simulink library "csu_und_unduplicate_lib"  (R2014b)
settings: Solver=ode45  SolverMode=SingleTasking  StartTime=0.0  StopTime=10.0  RelTol=1e-3
libraries: util_info_lib x1
settings Model: ExtModeAutoUpdateStatusClock=off  Creator=Administrator  LastModifiedBy=mstewart

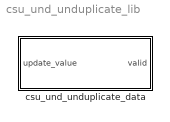
== system csu_und_unduplicate_lib ==
  csu_und_unduplicate_data : Subsystem  mask{initial_compare=0}
      mask prompts: initial_compare "initial comparison value"
      mask Display:
      | port_label('input',1,'update');
      | port_label('output',1','valid');

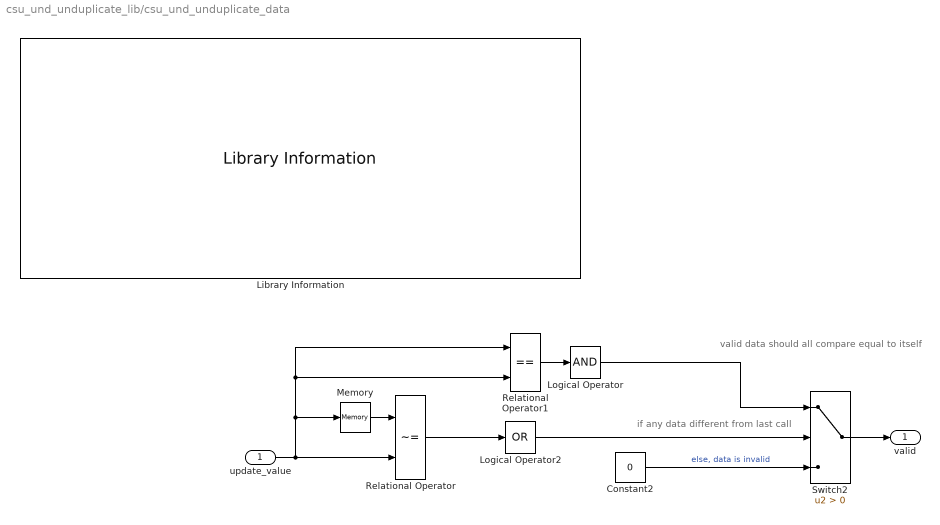
== system csu_und_unduplicate_lib/csu_und_unduplicate_data ==
  note: if any data different from last call
  note: valid data should all compare equal to itself
  update_value : Inport
  Constant2 : Constant  Value=0
  Library Information : util_info_lib/Library Information  owner='NONE'
  Logical Operator : Logic  Inputs=1  AllPortsSameDT=off  OutDataTypeStr=boolean
  Logical Operator2 : Logic  Operator=OR  Inputs=1  AllPortsSameDT=off  OutDataTypeStr=boolean
  Memory : Memory  X0=initial_compare  InheritSampleTime=on
  Relational Operator : RelationalOperator  Operator=~=  OutDataTypeStr=boolean
  Relational Operator1 : RelationalOperator  Operator===  OutDataTypeStr=boolean
  Switch2 : Switch  Criteria=u2 > Threshold
  valid : Outport  InitialOutput=1
  wires:
  Switch2/1 -> valid/1
  Logical Operator/1 -> Switch2/1
  Relational Operator1/1 -> Logical Operator/1
  update_value/1 -> Relational Operator/2, Memory/1, Relational Operator1/2, Relational Operator1/1
  Relational Operator/1 -> Logical Operator2/1
  Constant2/1 -> Switch2/3  "else, data is invalid"
  Memory/1 -> Relational Operator/1
  Logical Operator2/1 -> Switch2/2
